simulink model "OPAMPs"  (R2024a)
settings: Solver=VariableStepAuto  StartTime=0.0  StopTime=5  RelTol=1e-3
settings Model: Creator=Charles  LastModifiedBy=Racso
settings SolverCC: AlgebraicLoopSolver=TrustRegion
settings DataIOCC: ReturnWorkspaceOutputs=off
settings DebuggingCC: UnconnectedInputMsg=warning  UnconnectedOutputMsg=warning  UnconnectedLineMsg=warning  ArithmeticOperatorsInVariantConditions=warning
settings ModelReferenceCC: EnableRefExpFcnMdlSchedulingChecks=on
settings SFSimCC: SimUseLocalCustomCode=off  CustomCodeUndefinedFunction=UseInterfaceOnly
settings RTWCC: RTWUseLocalCustomCode=off  GPUComputeCapability=3.5

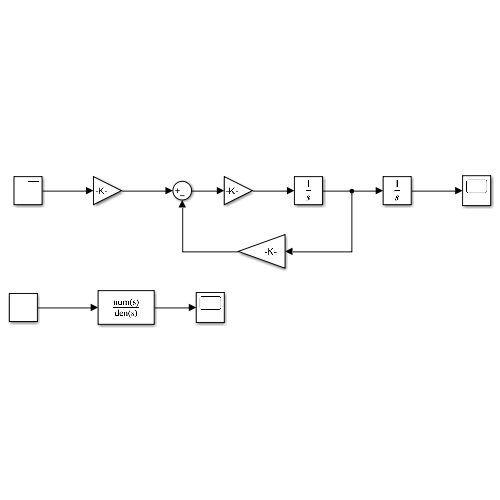
[thumbnail: Simulink's stored preview of the top-level diagram]
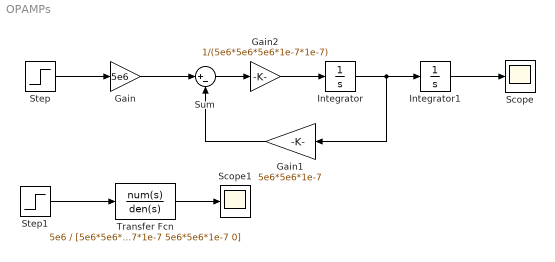
== system OPAMPs ==
  Gain : Gain  Gain=5e6
  Gain1 : Gain  Gain=5e6*5e6*1e-7
  Gain2 : Gain  Gain=1/(5e6*5e6*5e6*1e-7*1e-7)
  Integrator : Integrator
  Integrator1 : Integrator
  Scope : Scope
  Scope1 : Scope
  Step : Step  Time=0  After=5  SampleTime=0
  Step1 : Step  Time=0  After=5  SampleTime=0
  Sum : Sum  Inputs=|+-
  Transfer Fcn : TransferFcn  Numerator=5e6  Denominator=[5e6*5e6*5e6*1e-7*1e-7 5e6*5e6*1e-7 0]
  wires:
  Step/1 -> Gain/1
  Gain/1 -> Sum/1
  Integrator/1 -> Gain1/1, Integrator1/1
  Integrator1/1 -> Scope/1
  Gain1/1 -> Sum/2
  Sum/1 -> Gain2/1
  Gain2/1 -> Integrator/1
  Step1/1 -> Transfer Fcn/1
  Transfer Fcn/1 -> Scope1/1
